simulink model "Prueba2"  (R2023a)
settings: Solver=VariableStepAuto  StartTime=0.0  StopTime=10000  RelTol=1e-3
settings Model: Creator=laura  LastModifiedBy=laura

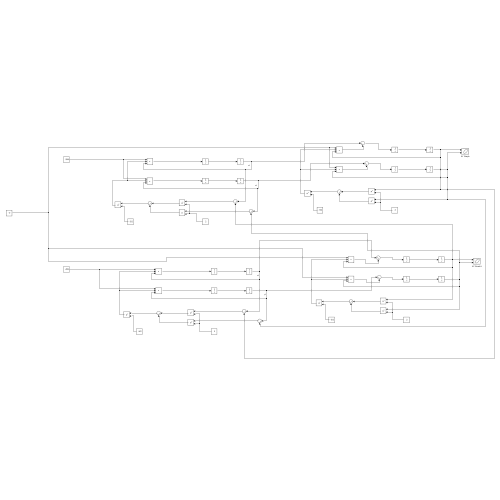
[thumbnail: Simulink's stored preview of the top-level diagram]
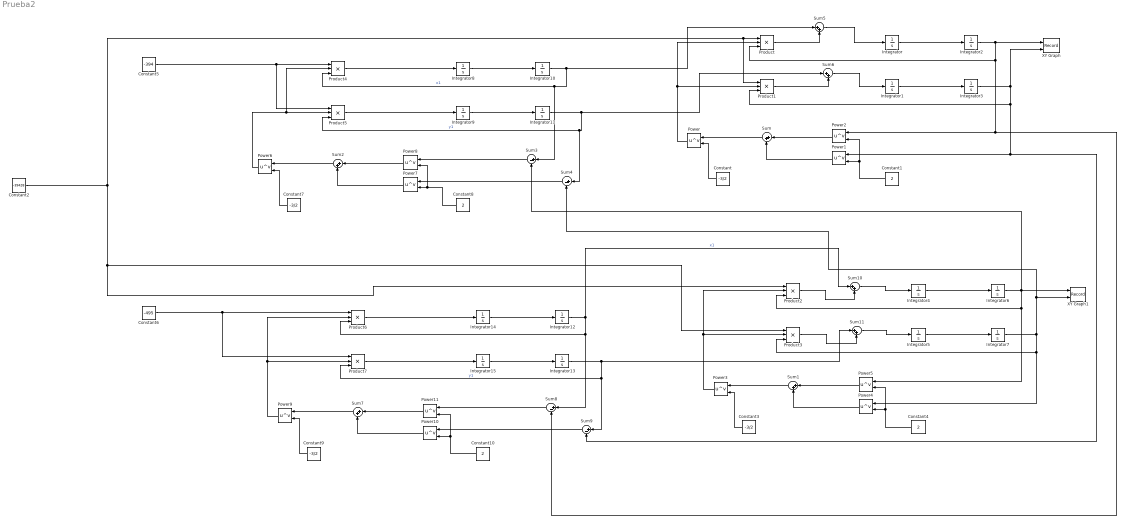
== system Prueba2 ==
  Constant{,3,7,9} (4 alike) : Constant  Value=-3/2
  Constant{1,4,8,10} (4 alike) : Constant  Value=2
  Constant2 : Constant  Value=-39428
  Constant5 : Constant  Value=-394
  Constant6 : Constant  Value=-495
  Integrator{,1,4..5,8..9,14..15} (8 alike) : Integrator  InitialCondition=-1
  Integrator{2,6,10,12} (4 alike) : Integrator
  Integrator11 : Integrator  InitialCondition=1000
  Integrator13 : Integrator  InitialCondition=1000
  Integrator3 : Integrator  InitialCondition=38700
  Integrator7 : Integrator  InitialCondition=38700
  Power{,1..11} (12 alike) : Math  Operator=pow
  Product{,1..7} (8 alike) : Product  Inputs=3
  Sum{,1..2,5..7,10..11} (8 alike) : Sum  Inputs=|++
  Sum{3..4,8..9} (4 alike) : Sum  Inputs=|+-
  XY Graph : Record  FileSettingsInternal="{\"entries\":[{\"content\":{\"excelSettings\":{\"content\":{},\"type\":\"Streamout.ExcelSettings\"}},\"type\":\"Streamout.FileSettingStorage\",\"uuid\":\"889edef3-f547-4079-9f63-05b3711ec7f4\"}],\"packageUris\":[\"http://schema.mathworks.com/mf0/streamout_blocks/R2020a\"],\"version\":\"1.0\"}"  Layout=[1 1]  SignalsInternal="{\"entries\":[{\"content\":{\"signals\":[{\"content\":{\"blockPath\":[\"Prueba2/XY Graph\"],\"dimensions\":[1],\"domain\":\"Prueba2/XY Graph\",\"lineColor\":\"#a2142f\",\"plots\":[1],\"port\":1,\"signalID\":25,\"signalName\":\"Integrator2\"},\"type\":\"RecordBlkView.Signal\",\"uuid\":\"35a284fe-76d7-4d90-af77-c383a435fd92\"},{\"content\":{\"blockPath\":[\"Prueba2/XY Graph\"],\"dimensions\":[1],\"domain\":\"Prueba2/XY Graph\",\"lineColor\":\"#139fff\",\"plots\":[1],\"port\":2,\"signalID\":28,\"signalName\":\"Integrator3\"},\"type\":\"RecordBlkView.Signal\",\"uuid\":\"eee25935-15f1-469f-a772-0a58d62109b6\"}]},\"type\":\"RecordBlkView.InputSignals\",\"uuid\":\"56407368-544b-48f6-951e-c826b6fa65f6\"}],\"packageUris\":[\"http://schema.mathworks.com/mf0/streamout_blocks/R2020a\"],\"version\":\"1.0\"}"  VisualizationBindings="{\"xyplotplugin\":{\"info\":[{\"series\":[{\"bindingParametersList\":[{\"parameter\":\"X-Axis\",\"signalID\":25,\"signalName\":\"Integrator2\"},{\"parameter\":\"Y-Axis\",\"signalID\":28,\"signalName\":\"Integrator3\"}],\"seriesID\":45781}],\"subplotID\":1}]}}"  CompatibilityTag=XY
  XY Graph1 : Record  FileSettingsInternal="{\"entries\":[{\"content\":{\"excelSettings\":{\"content\":{},\"type\":\"Streamout.ExcelSettings\"}},\"type\":\"Streamout.FileSettingStorage\",\"uuid\":\"e0429362-7c1c-425f-abb2-55b1d682c498\"}],\"packageUris\":[\"http://schema.mathworks.com/mf0/streamout_blocks/R2020a\"],\"version\":\"1.0\"}"  Layout=[1 1]  SignalsInternal="{\"entries\":[{\"content\":{\"signals\":[{\"content\":{\"blockPath\":[\"Prueba2/XY Graph1\"],\"dimensions\":[1],\"domain\":\"Prueba2/XY Graph1\",\"lineColor\":\"#a2142f\",\"port\":1,\"signalID\":17,\"signalName\":\"Integrator6\"},\"type\":\"RecordBlkView.Signal\",\"uuid\":\"d1edd32c-00c9-4833-8f47-9970b8fe1f08\"},{\"content\":{\"blockPath\":[\"Prueba2/XY Graph1\"],\"dimensions\":[1],\"domain\":\"Prueba2/XY Graph1\",\"lineColor\":\"#139fff\",\"port\":2,\"signalID\":20,\"signalName\":\"Integrator7\"},\"type\":\"RecordBlkView.Signal\",\"uuid\":\"fc945eec-82b7-437f-a2da-334a543ac4fc\"}]},\"type\":\"RecordBlkView.InputSignals\",\"uuid\":\"0a6ded57-a2da-40f7-b765-29d7d008ebad\"}],\"packageUris\":[\"http://schema.mathworks.com/mf0/streamout_blocks/R2020a\"],\"version\":\"1.0\"}"  VisualizationBindings="{\"xyplotplugin\":{\"info\":[{\"series\":[],\"subplotID\":1}]}}"  CompatibilityTag=XY
  wires:
  Constant/1 -> Power/2
  Integrator1/1 -> Integrator3/1
  Sum/1 -> Power/1
  Integrator/1 -> Integrator2/1
  Constant1/1 -> Power2/2, Power1/2
  Integrator2/1 -> Power2/1, Sum8/2, Product/3, XY Graph/1
  Power/1 -> Product1/2, Product/2
  Constant2/1 -> Product1/1, Product/1, Product2/1, Product3/1
  Integrator3/1 -> XY Graph/2, Sum9/2, Power1/1, Product1/3
  Power2/1 -> Sum/1
  Power1/1 -> Sum/2
  Sum1/1 -> Power3/1
  Constant4/1 -> Power5/2, Power4/2
  Integrator5/1 -> Integrator7/1
  Integrator6/1 -> XY Graph1/1, Power5/1, Product2/3, Sum3/2
  Power5/1 -> Sum1/1
  Power4/1 -> Sum1/2
  Constant3/1 -> Power3/2
  Integrator7/1 -> Sum4/2, XY Graph1/2, Power4/1, Product3/3
  Power3/1 -> Product3/2, Product2/2
  Integrator4/1 -> Integrator6/1
  Product5/1 -> Integrator9/1
  Sum2/1 -> Power6/1
  Constant8/1 -> Power8/2, Power7/2
  Integrator9/1 -> Integrator11/1
  Integrator10/1 -> Sum3/1, Product4/3, Sum5/1  "x1"
  Product4/1 -> Integrator8/1
  Power8/1 -> Sum2/1
  Power7/1 -> Sum2/2
  Constant7/1 -> Power6/2
  Integrator11/1 -> Sum4/1, Product5/3, Sum6/1  "y1"
  Power6/1 -> Product5/2, Product4/2
  Integrator8/1 -> Integrator10/1
  Constant5/1 -> Product5/1, Product4/1
  Sum3/1 -> Power8/1
  Sum4/1 -> Power7/1
  Product/1 -> Sum5/2
  Sum5/1 -> Integrator/1
  Product1/1 -> Sum6/2
  Sum6/1 -> Integrator1/1
  Power9/1 -> Product7/2, Product6/2
  Sum9/1 -> Power10/1
  Constant10/1 -> Power11/2, Power10/2
  Integrator13/1 -> Sum11/1, Sum9/1, Product7/3  "y1"
  Product6/1 -> Integrator14/1
  Power10/1 -> Sum7/2
  Sum7/1 -> Power9/1
  Product7/1 -> Integrator15/1
  Constant9/1 -> Power9/2
  Power11/1 -> Sum7/1
  Integrator14/1 -> Integrator12/1
  Sum8/1 -> Power11/1
  Integrator15/1 -> Integrator13/1
  Integrator12/1 -> Sum8/1, Product6/3, Sum10/1  "x1"
  Constant6/1 -> Product7/1, Product6/1
  Product2/1 -> Sum10/2
  Sum10/1 -> Integrator4/1
  Product3/1 -> Sum11/2
  Sum11/1 -> Integrator5/1
